simulink model "exercise13"  (R2017a)
settings: Solver=VariableStepAuto  StartTime=0.0  StopTime=25  RelTol=1e-3
values from neighbouring files (symbols this model uses):
  b = 1    [assignment1.m]
  K = 167    [assignment1.m]
  N = 2    [assignment1.m]
settings Model: Creator=viktor  LastModifiedBy=viktor

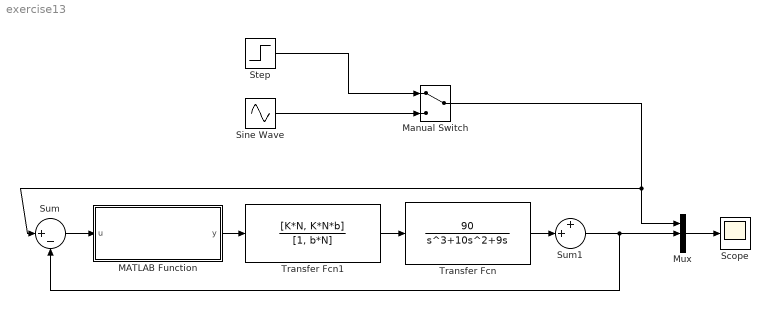
== system exercise13 ==
  MATLAB Function : MATLAB Function  TreatAsAtomicUnit=on
  Manual Switch : ManualSwitch
  Mux : Mux  Inputs=3
  Scope : Scope
  Sine Wave : Sin  Amplitude=.01  Frequency=3  SampleTime=0
  Step : Step  SampleTime=0
  Sum : Sum  Inputs=|+-
  Sum1 : Sum  Inputs=++|
  Transfer Fcn : TransferFcn  Numerator=[90]  Denominator=[1 10 9 0]
  Transfer Fcn1 : TransferFcn  Numerator=[K*N, K*N*b]  Denominator=[1, b*N]
  wires:
  Sum/1 -> MATLAB Function/1(u)
  Mux/1 -> Scope/1
  Transfer Fcn/1 -> Sum1/2
  Sum1/1 -> Sum/2, Mux/2
  Sine Wave/1 -> Manual Switch/2
  Step/1 -> Manual Switch/1
  Manual Switch/1 -> Mux/1, Sum/1
  Transfer Fcn1/1 -> Transfer Fcn/1
  MATLAB Function/1(y) -> Transfer Fcn1/1

== matlab function exercise13/MATLAB Function ==
  data: u input; y output
function y = relay_with_deadzone(u)
    if u <= -.2
        y = -1;
    elseif u >= .2
        y = 1;
    else
        y = 0;
    end
end
